simulink model "kinsim_2link_planar"  (R2020a)
settings: Solver=ode3  StartTime=0.0  StopTime=10.0  FixedStep=0.05  RelTol=1e-3
values from neighbouring files (symbols this model uses):
  dh = [0.337,0,-pi/2; 0,0.21,0; 0,0,-pi/2; 0.268,0,pi/2; 0,0,-pi/2; 0.174,0,0]    [provacinematica.m]
libraries: robotlib x12
settings Model: Creator=ROS_PO  LastModifiedBy=luca
settings OptimizationCC: EnhancedBackFolding=on  PassReuseOutputArgsAs=Individual arguments  ZeroExternalMemoryAtStartup=off  ZeroInternalMemoryAtStartup=off  MaxStackSize=64  OptimizeBlockOrder=speed  DifferentSizesBufferReuse=on  OptimizationCustomize=off  EfficientTunableParamExpr=on
settings DebuggingCC: ParameterTunabilityLossMsg=error
settings HardwareCC: ProdBitPerPointer=32  ProdBitPerSizeT=32  ProdBitPerPtrDiffT=32  ProdLargestAtomicFloat=None  ProdIntDivRoundTo=Undefined  ProdEndianess=Unspecified  ProdWordSize=32  ProdHWDeviceType=Generic->Unspecified (assume 32-bit Generic)
settings RTWCC: SystemTargetFile=ert.tlc  HardwareBoard=Robot Operating System (ROS)  TemplateMakefile=ert_default_tmf  GenerateReport=on  Toolchain=Catkin  IncludeHyperlinkInReport=on  LaunchReport=on  TargetLang=C++  GenerateTraceInfo=on  GenerateTraceReport=on  GenerateTraceReportSl=on  GenerateTraceReportSf=on  GenerateTraceReportEml=on
settings CodeAppCC: ForceParamTrailComments=on  IgnoreCustomStorageClasses=off  OperatorAnnotations=on  SimulinkDataObjDesc=on  SFDataObjDesc=on  InsertBlockDesc=on
settings ERTTargetCC: SupportContinuousTime=on  SupportVariableSizeSignals=on

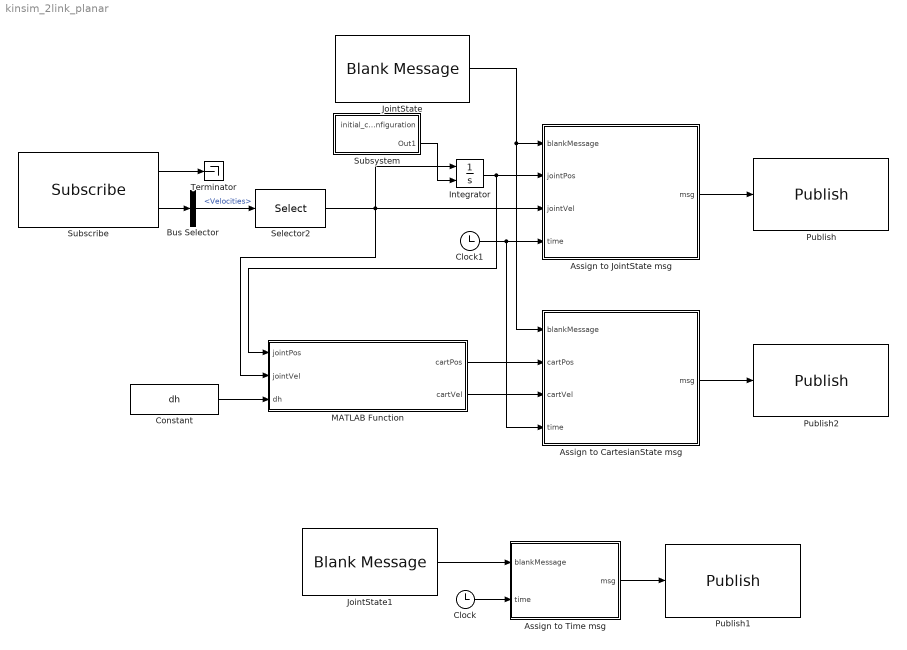
== system kinsim_2link_planar ==
  Assign to CartesianState msg : MATLAB Function  TreatAsAtomicUnit=on
  Assign to JointState msg : MATLAB Function  TreatAsAtomicUnit=on
  Assign to Time msg : MATLAB Function  TreatAsAtomicUnit=on
  Bus Selector : BusSelector  OutputSignals=Velocities
  Clock : Clock
  Clock1 : Clock
  Constant : Constant  Value=dh
  Integrator : Integrator  InitialConditionSource=external  InitialCondition=[0,0]
  JointState : robotlib/Blank Message  messageClass=Message  entityType=sensor_msgs/JointState  messageType=sensor_msgs/JointState  SampleTime=inf
  JointState1 : robotlib/Blank Message  messageClass=Message  entityType=rosgraph_msgs/Clock  messageType=rosgraph_msgs/Clock  SampleTime=inf
  MATLAB Function : MATLAB Function  TreatAsAtomicUnit=on
  Publish : robotlib/Publish  topicSource=Specify your own  topic=/joint_states  messageType=sensor_msgs/JointState  messageQueueLength=1
  Publish1 : robotlib/Publish  topicSource=Specify your own  topic=/clock  messageType=rosgraph_msgs/Clock  messageQueueLength=1
  Publish2 : robotlib/Publish  topicSource=Specify your own  topic=/cartesian_states  messageType=sensor_msgs/JointState  messageQueueLength=1
  Selector2 : Selector  IndexOptions=Starting index (dialog)  Indices=[1]  OutputSizes=6
  Subscribe : robotlib/Subscribe  topicSource=Specify your own  topic=/joint_trajectory  messageType=trajectory_msgs/JointTrajectoryPoint  sampleTime=-1  messageQueueLength=1
  Subsystem : Subsystem
  Terminator : Terminator
  wires:
  Subscribe/1 -> Terminator/1
  Subscribe/2 -> Bus Selector/1
  Bus Selector/1 -> Selector2/1  "<Velocities>"
  Integrator/1 -> MATLAB Function/1(jointPos), Assign to JointState msg/2(jointPos)
  Selector2/1 -> Assign to JointState msg/3(jointVel), MATLAB Function/2(jointVel), Integrator/1
  Assign to JointState msg/1(msg) -> Publish/1
  JointState/1 -> Assign to CartesianState msg/1(blankMessage), Assign to JointState msg/1(blankMessage)
  JointState1/1 -> Assign to Time msg/1(blankMessage)
  Clock/1 -> Assign to Time msg/2(time)
  Assign to Time msg/1(msg) -> Publish1/1
  Clock1/1 -> Assign to CartesianState msg/4(time), Assign to JointState msg/4(time)
  MATLAB Function/1(cartPos) -> Assign to CartesianState msg/2(cartPos)
  MATLAB Function/2(cartVel) -> Assign to CartesianState msg/3(cartVel)
  Assign to CartesianState msg/1(msg) -> Publish2/1
  Constant/1 -> MATLAB Function/3(dh)
  Subsystem/2(Out1) -> Integrator/2

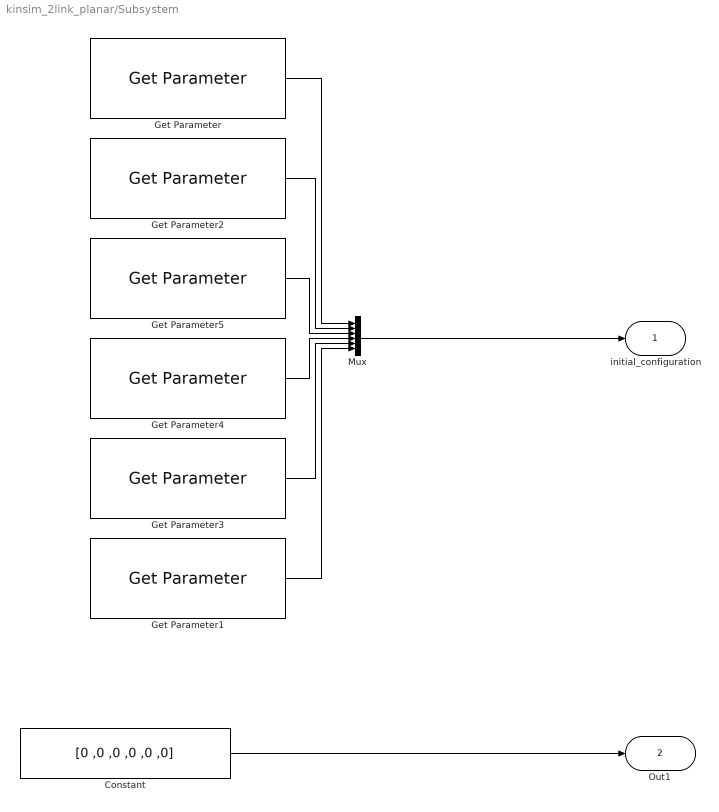
== system kinsim_2link_planar/Subsystem ==
  Constant : Constant  Value=[0 ,0 ,0 ,0 ,0 ,0]
  Get Parameter : robotlib/Get Parameter  ParameterSource=Specify your own  ParameterName=/kinsim_2link_planar/q1_initial  ParameterType=double  ParameterMaxArrayLength=16  ParameterInitialValue=pi/4  SampleTime=-1  ShowErrorCodeOutput=off  ModelName=kinsim_2link_planar  BlockId=ParamGet_kinsim_2link_planar_61
      settings: SourceProductBaseCode=RR
  Get Parameter1 : robotlib/Get Parameter  ParameterSource=Specify your own  ParameterName=/kinsim_2link_planar/q6_initial  ParameterType=double  ParameterMaxArrayLength=16  ParameterInitialValue=-pi/4  SampleTime=-1  ShowErrorCodeOutput=off  ModelName=kinsim_2link_planar  BlockId=ParamGet_kinsim_2link_planar_65
      settings: SourceProductBaseCode=RR
  Get Parameter2 : robotlib/Get Parameter  ParameterSource=Specify your own  ParameterName=/kinsim_2link_planar/q2_initial  ParameterType=double  ParameterMaxArrayLength=16  ParameterInitialValue=-pi/4  SampleTime=-1  ShowErrorCodeOutput=off  ModelName=kinsim_2link_planar  BlockId=ParamGet_kinsim_2link_planar_85
      settings: SourceProductBaseCode=RR
  Get Parameter3 : robotlib/Get Parameter  ParameterSource=Specify your own  ParameterName=/kinsim_2link_planar/q5_initial  ParameterType=double  ParameterMaxArrayLength=16  ParameterInitialValue=-pi/4  SampleTime=-1  ShowErrorCodeOutput=off  ModelName=kinsim_2link_planar  BlockId=ParamGet_kinsim_2link_planar_86
      settings: SourceProductBaseCode=RR
  Get Parameter4 : robotlib/Get Parameter  ParameterSource=Specify your own  ParameterName=/kinsim_2link_planar/q4_initial  ParameterType=double  ParameterMaxArrayLength=16  ParameterInitialValue=-pi/4  SampleTime=-1  ShowErrorCodeOutput=off  ModelName=kinsim_2link_planar  BlockId=ParamGet_kinsim_2link_planar_87
      settings: SourceProductBaseCode=RR
  Get Parameter5 : robotlib/Get Parameter  ParameterSource=Specify your own  ParameterName=/kinsim_2link_planar/q3_initial  ParameterType=double  ParameterMaxArrayLength=16  ParameterInitialValue=-pi/4  SampleTime=-1  ShowErrorCodeOutput=off  ModelName=kinsim_2link_planar  BlockId=ParamGet_kinsim_2link_planar_88
      settings: SourceProductBaseCode=RR
  Mux : Mux  Inputs=6
  initial_configuration : Outport
  Out1 : Outport  Port=2
  wires:
  Mux/1 -> initial_configuration/1
  Get Parameter/1 -> Mux/1
  Get Parameter1/1 -> Mux/6
  Get Parameter2/1 -> Mux/2
  Get Parameter4/1 -> Mux/4
  Get Parameter3/1 -> Mux/5
  Get Parameter5/1 -> Mux/3
  Constant/1 -> Out1/1

== matlab function kinsim_2link_planar/Assign to Time msg ==
  data: blankMessage input; msg output Bus: SL_Bus_kinsim_2link_planar_rosgraph_msgs_Clock; time input
function msg = assign_Time(blankMessage,time)
%#codegen

% Assign the output message to be the same with input blank message
msg = blankMessage;

% Convert and set time
msg.Clock_.Sec  = fix(time);
msg.Clock_.Nsec = fix((time-fix(time))*1e9);

== matlab function kinsim_2link_planar/Assign to JointState msg ==
  data: blankMessage input; msg output Bus: SL_Bus_kinsim_2link_planar_sensor_msgs_JointState; jointPos input; jointVel input; time input
function msg = assign_JointState(blankMessage,jointPos,jointVel,time)
%#codegen

% Assign the output message to be the same with input blank message
msg = blankMessage;

% Initialize time stamp
msg.Header.Stamp.Sec  = fix(time);
msg.Header.Stamp.Nsec = fix((time-fix(time))*1e9);

% Set the number of strings in the string array, and joint positions/velocities in the position/velocity array
numJoints = length(jointPos);
msg.Name_SL_Info.CurrentLength = uint32(numJoints);
msg.Position_SL_Info.CurrentLength = uint32(numJoints);
msg.Velocity_SL_Info.CurrentLength = uint32(numJoints);

% Set the individual components in the message arrays
strArrayToAssign = {'joint_1', 'joint_2', 'joint_3', 'joint_4', 'joint_5', 'joint_6'};

for idx=1:numJoints
    str = strArrayToAssign{idx};
    strLength = length(str);
    msg.Name(idx).Data(1:strLength) = uint8(str);
    msg.Name(idx).Data_SL_Info.CurrentLength = uint32(strLength);

    msg.Position(idx) = jointPos(idx);
    msg.Velocity(idx) = jointVel(idx);
end

== matlab function kinsim_2link_planar/MATLAB Function ==
  data: jointPos input; cartPos output; jointVel input; cartVel output; dh input
function [cartPos, cartVel] = forward_kinematics_2link(jointPos,jointVel,dh)
%dh è una matrice di denavit hart...
%dh=[0.337,0,-pi/2; 0,0.21,0; 0,0,-pi/2; 0.268,0,pi/2; 0,0,-pi/2; 0.174,0,0];

cartPos = zeros(6,1);
cartVel = zeros(6,1);
A=zeros(4,4,6);
T=zeros(4,4,6);
%jointPos = [0,-pi/2,-pi/2,-pi,-pi,0];


for i=1:6
 A(:,:,i) = [ cos(jointPos(i)),-sin(jointPos(i))*cos(dh(i,3)), sin(jointPos(i))*sin(dh(i,3)),dh(i,2)*cos(jointPos(i));
              sin(jointPos(i)), cos(jointPos(i))*cos(dh(i,3)),-cos(jointPos(i))*sin(dh(i,3)),dh(i,2)*sin(jointPos(i));
              0,                        sin(dh(i,3)),               cos(dh(i,3)),                   dh(i,1);
              0,                            0,                           0,                            1];
end
T(:,:,1) = A(:,:,1);
for i=2:6
    T(:,:,i) = T(:,:,i-1)*A(:,:,i);
end
cartPos(1:3) = T(1:3,4,6);
cartPos(4:6) = rotm2eul(T(1:3,1:3,6));

J = zeros(6,6);
J(1:3,1) = cross([0,0,1],T(1:3,4,6));
J(4:6,1) = [0;0;1];
for i = 2:6
    J(1:3,i) = cross(T(1:3,3,i-1),T(1:3,4,6)-T(1:3,4,i-1));
    J(4:6,i) = T(1:3,3,i-1);
end

R = [0,-sin(cartPos(4)),cos(cartPos(4))*sin(cartPos(5));
     0,cos(cartPos(4)), sin(cartPos(4))*sin(cartPos(5));
     1,     0,              cos(cartPos(5))];
 
cartVel = J*jointVel;
cartVel(4:6)=R*cartVel(4:6);

== matlab function kinsim_2link_planar/Assign to CartesianState msg ==
  data: blankMessage input; msg output Bus: SL_Bus_kinsim_2link_planar_sensor_msgs_JointState; cartPos input; cartVel input; time input
function msg = assign_CartesianState(blankMessage,cartPos,cartVel,time)
%#codegen

% Assign the output message to be the same with input blank message
msg = blankMessage;

% Initialize time stamp
msg.Header.Stamp.Sec  = fix(time);
msg.Header.Stamp.Nsec = fix((time-fix(time))*1e9);

% Set the number of strings in the string array, and joint positions/velocities in the position/velocity array
numCoordinates = length(cartPos);
msg.Name_SL_Info.CurrentLength = uint32(numCoordinates);
msg.Position_SL_Info.CurrentLength = uint32(numCoordinates);
msg.Velocity_SL_Info.CurrentLength = uint32(numCoordinates);

% Set the individual components in the message arrays
strArrayToAssign = {'joint_1', 'joint_2', 'joint_3', 'joint_4', 'joint_5', 'joint_6'};

for idx=1:numCoordinates
    str = strArrayToAssign{idx};
    strLength = length(str);
    msg.Name(idx).Data(1:strLength) = uint8(str);
    msg.Name(idx).Data_SL_Info.CurrentLength = uint32(strLength);

    msg.Position(idx) = cartPos(idx);
    msg.Velocity(idx) = cartVel(idx);
end
